simulink model "sampleModel1938"  (R2023a)
settings: Solver=VariableStepAuto  StartTime=0.0  StopTime=10.0  RelTol=1e-3
libraries: hdlsllib x3
settings Model: Creator=user1  LastModifiedBy=user1

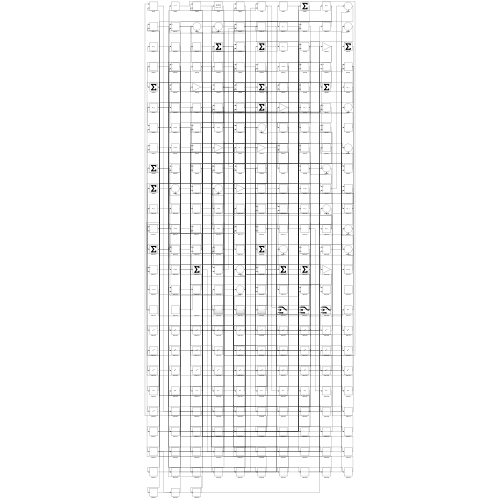
[thumbnail: Simulink's stored preview of the top-level diagram]
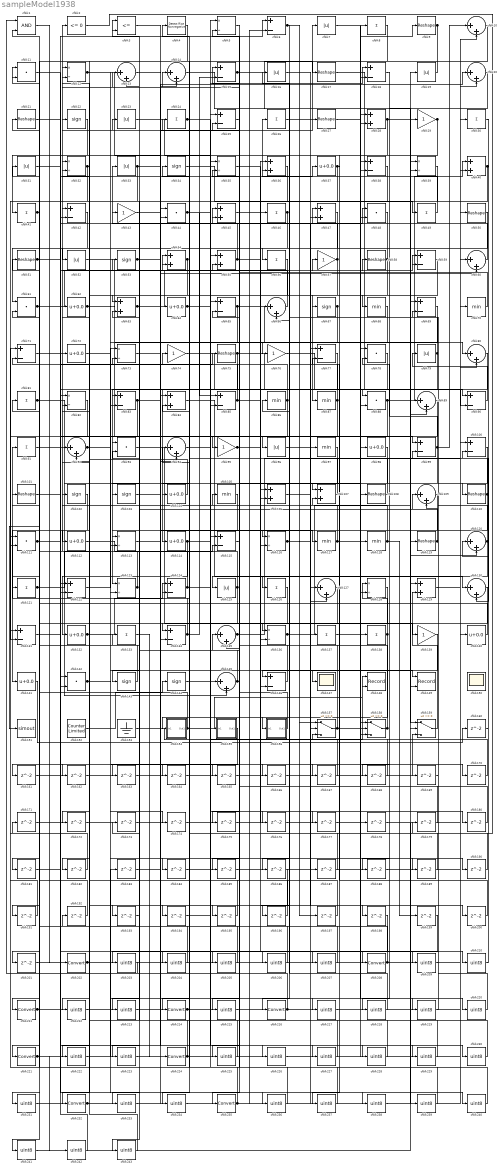
== system sampleModel1938 ==
  cfblk1 : Logic  AllPortsSameDT=off  OutDataTypeStr=boolean
  cfblk{10,13..14,20,60,66,80,89,92,94,109,120,127,130,135,145} (16 alike) : Sum  Inputs=|++
  cfblk{6,15,18,25,38,42,59,65,69,71,77,83,85,90,99..100,115,122,124,131,134,146} (22 alike) : Sum  Inputs=+-
  cfblk{9,17,21,27,50..51,58,75,101,108,110,119} (12 alike) : Reshape
  cfblk{22,34,53,67,102..103,143..144} (8 alike) : Signum
  cfblk{37,62,64,72,98,104,112,114,132,140..141} (11 alike) : Bias  Bias=0.0  SaturateOnIntegerOverflow=off
  cfblk{68,70,86..87,97,105,117..118} (8 alike) : MinMax
  cfblk{28,36,40,45,47,54..55,63,84,106..107,129} (12 alike) : Sum
  cfblk{11,44,48,61,78,88,93,111,142} (9 alike) : DotProduct  OutDataTypeStr=Inherit: Inherit via internal rule
  cfblk{5,12,32,35,39,73,82,113,116,123,128,136} (12 alike) : Product  Inputs=*/  RndMeth=Zero  SaturateOnIntegerOverflow=on
  cfblk{8,24,26,30,41,46,49,56,81,91,121,126,133,137..138} (15 alike) : Sum  Inputs=+
  cfblk{7,16,19,23,31,33,52,79,96,125} (10 alike) : Abs  SaturateOnIntegerOverflow=off
  cfblk{29,43,57,74,76,95,139} (7 alike) : Gain
  cfblk147 : Scope
  cfblk148 : Record  FileSettingsInternal="{\"entries\":[{\"content\":{\"excelSettings\":{\"content\":{},\"type\":\"Streamout.ExcelSettings\"}},\"type\":\"Streamout.FileSettingStorage\",\"uuid\":\"\"}],\"packageUris\":[\"http:\\/\\/schema.mathworks.com\\/mf0\\/streamout_blocks\\/R2020a\"],\"version\":\"1.0\"}"  Layout=[1 1]  SignalsInternal="{\"entries\":[{\"content\":{\"signals\":[{\"content\":{\"blockPath\":[],\"dimensions\":[1],\"domain\":\"\",\"lineColor\":\"#a2142f\",\"plots\":[1],\"port\":1,\"signalID\":5311,\"signalName\":\"XY Graph:1\"},\"type\":\"RecordBlkView.Signal\",\"uuid\":\"\"},{\"content\":{\"blockPath\":[],\"dimensions\":[1],\"domain\":\"\",\"lineColor\":\"#139fff\",\"plots\":[1],\"port\":2,\"signalID\":5314,\"signalName\":\"XY Graph:2\"},\"type\":\"RecordBlkView.Signal\",\"uuid\":\"\"}]},\"type\":\"RecordBlkView.InputSignals\",\"uuid\":\"\"}],\"packageUris\":[\"http:\\/\\/schema.mathworks.com\\/mf0\\/streamout_blocks\\/R2020a\"],\"version\":\"1.0\"}"  VisualizationBindings="{\"xyplotplugin\":{\"info\":[{\"series\":[{\"bindingParametersList\":[{\"parameter\":\"X-Axis\",\"signalID\":5311,\"signalName\":\"XY Graph:1\"},{\"parameter\":\"Y-Axis\",\"signalID\":5314,\"signalName\":\"XY Graph:2\"}],\"seriesID\":33209}],\"subplotID\":1}]}}"  CompatibilityTag=XY  st=-1
  cfblk149 : Record  FileSettingsInternal="{\"entries\":[{\"content\":{\"excelSettings\":{\"content\":{},\"type\":\"Streamout.ExcelSettings\"}},\"type\":\"Streamout.FileSettingStorage\",\"uuid\":\"\"}],\"packageUris\":[\"http:\\/\\/schema.mathworks.com\\/mf0\\/streamout_blocks\\/R2020a\"],\"version\":\"1.0\"}"  Layout=[1 1]  SignalsInternal="{\"entries\":[{\"content\":{\"signals\":[{\"content\":{\"blockPath\":[],\"dimensions\":[1],\"domain\":\"\",\"lineColor\":\"#a2142f\",\"plots\":[1],\"port\":1,\"signalID\":5319,\"signalName\":\"XY Graph:1\"},\"type\":\"RecordBlkView.Signal\",\"uuid\":\"\"},{\"content\":{\"blockPath\":[],\"dimensions\":[1],\"domain\":\"\",\"lineColor\":\"#139fff\",\"plots\":[1],\"port\":2,\"signalID\":5322,\"signalName\":\"XY Graph:2\"},\"type\":\"RecordBlkView.Signal\",\"uuid\":\"\"}]},\"type\":\"RecordBlkView.InputSignals\",\"uuid\":\"\"}],\"packageUris\":[\"http:\\/\\/schema.mathworks.com\\/mf0\\/streamout_blocks\\/R2020a\"],\"version\":\"1.0\"}"  VisualizationBindings="{\"xyplotplugin\":{\"info\":[{\"series\":[{\"bindingParametersList\":[{\"parameter\":\"X-Axis\",\"signalID\":5319,\"signalName\":\"XY Graph:1\"},{\"parameter\":\"Y-Axis\",\"signalID\":5322,\"signalName\":\"XY Graph:2\"}],\"seriesID\":898}],\"subplotID\":1}]}}"  CompatibilityTag=XY  st=-1
  cfblk150 : Scope
      settings: Floating=on
  cfblk151 : ToWorkspace  VariableName=simout  SaveFormat=Timeseries  SampleTime=-1
  cfblk152 : hdlsllib/Sources/Counter Limited  uplimit=7  tsamp=-1
  cfblk153 : Ground
  cfblk154 : Subsystem
      settings: LibrarySourceBlock=|
      | hdlsllib/Ports &
      | Subsystems/Subsystem
  cfblk155 : Subsystem
      settings: LibrarySourceBlock=|
      | hdlsllib/Ports &
      | Subsystems/Subsystem
  cfblk156 : Subsystem
      settings: LibrarySourceBlock=|
      | hdlsllib/Ports &
      | Subsystems/Subsystem
  cfblk157 : Switch  SaturateOnIntegerOverflow=off  InputSameDT=off
  cfblk158 : Switch  SaturateOnIntegerOverflow=off  InputSameDT=off
  cfblk159 : Switch  SaturateOnIntegerOverflow=off  InputSameDT=off
  cfblk{160..201} (42 alike) : Delay  SampleTime=1
  cfblk2 : hdlsllib/Logic and Bit Operations/Compare To Zero  relop=<=  OutDataTypeStr=boolean
  cfblk{202,208,211,214,216,221,224,232,235} (9 alike) : DataTypeConversion  SaturateOnIntegerOverflow=off  RndMeth=Floor
  cfblk{203..207,209..210,212..213,215,217..220,222..223,225..231,233..234,236..243} (33 alike) : DataTypeConversion  OutDataTypeStr=uint8  SaturateOnIntegerOverflow=off  RndMeth=Floor
  cfblk3 : RelationalOperator  Operator=<=  OutDataTypeStr=boolean  InputSameDT=off
  cfblk4 : hdlsllib/Logic and Bit Operations/Detect Rise Nonnegative  vinit=0  OutDataTypeStr=boolean
  wires:
  cfblk116/1 -> cfblk157/1, cfblk190/1
  cfblk17/1 -> cfblk90/1
  cfblk55/1 -> cfblk33/1, cfblk200/1
  cfblk66/1 -> cfblk2/1
  cfblk138/1 -> cfblk128/1, cfblk234/1
  cfblk102/1 -> cfblk141/1
  cfblk118/1 -> cfblk42/1, cfblk199/1
  cfblk46/1 -> cfblk194/1, cfblk195/1
  cfblk19/1 -> cfblk96/1
  cfblk133/1 -> cfblk224/1
  cfblk26/1 -> cfblk7/1
  cfblk80/1 -> cfblk123/1
  cfblk57/1 -> cfblk87/1, cfblk85/2, cfblk45/2
  cfblk153/1 -> cfblk148/1
  cfblk33/1 -> cfblk52/1, cfblk60/2
  cfblk22/1 -> cfblk41/1
  cfblk25/1 -> cfblk235/1
  cfblk24/1 -> cfblk180/1, cfblk207/1
  cfblk41/1 -> cfblk151/1, cfblk11/1
  cfblk84/1 -> cfblk130/1
  cfblk40/1 -> cfblk130/2, cfblk76/1
  cfblk146/1 -> cfblk22/1
  cfblk152/1 -> cfblk144/1
  cfblk51/1 -> cfblk90/2, cfblk59/2
  cfblk127/1 -> cfblk232/1
  cfblk81/1 -> cfblk145/2, cfblk227/1
  cfblk134/1 -> cfblk91/1, cfblk15/2
  cfblk27/1 -> cfblk138/1
  cfblk88/1 -> cfblk40/1, cfblk134/2
  cfblk96/1 -> cfblk48/1
  cfblk156/1(Out1) -> cfblk54/1
  cfblk124/1 -> cfblk3/1, cfblk228/1
  cfblk114/1 -> cfblk132/1, cfblk57/1
  cfblk131/1 -> cfblk72/1
  cfblk4/1 -> cfblk121/1
  cfblk9/1 -> cfblk95/1, cfblk182/1
  cfblk79/1 -> cfblk43/1, cfblk168/1, cfblk243/1
  cfblk8/1 -> cfblk214/1
  cfblk37/1 -> cfblk47/2, cfblk237/1
  cfblk140/1 -> cfblk101/1
  cfblk135/1 -> cfblk30/1, cfblk139/1
  cfblk21/1 -> cfblk99/1
  cfblk87/1 -> cfblk66/2, cfblk215/1
  cfblk48/1 -> cfblk156/1(In1)
  cfblk77/1 -> cfblk93/1
  cfblk129/1 -> cfblk70/1
  cfblk137/1 -> cfblk9/1
  cfblk61/1 -> cfblk58/1, cfblk6/1
  cfblk42/1 -> cfblk61/1
  cfblk157/1 -> cfblk53/1, cfblk219/1
  cfblk154/1(Out1) -> cfblk148/2, cfblk31/1
  cfblk125/1 -> cfblk21/1, cfblk142/2
  cfblk14/1 -> cfblk98/1
  cfblk110/1 -> cfblk113/1, cfblk84/2
  cfblk36/1 -> cfblk103/1
  cfblk12/1 -> cfblk44/2, cfblk165/1
  cfblk104/1 -> cfblk12/1
  cfblk89/1 -> cfblk221/1
  cfblk50/1 -> cfblk216/1
  cfblk58/1 -> cfblk56/1, cfblk147/1
  cfblk117/1 -> cfblk4/1, cfblk16/1, cfblk149/1
  cfblk38/1 -> cfblk211/1
  cfblk99/1 -> cfblk107/1, cfblk78/2, cfblk10/1
  cfblk34/1 -> cfblk49/1
  cfblk28/1 -> cfblk120/2, cfblk122/2
  cfblk93/1 -> cfblk136/1
  cfblk63/1 -> cfblk19/1, cfblk116/2
  cfblk123/1 -> cfblk102/1, cfblk32/1
  cfblk73/1 -> cfblk27/1
  cfblk91/1 -> cfblk128/2
  cfblk75/1 -> cfblk114/1, cfblk158/3, cfblk149/2
  cfblk23/1 -> cfblk155/1(In1)
  cfblk54/1 -> cfblk112/1, cfblk233/1
  cfblk52/1 -> cfblk118/1
  cfblk1/1 -> cfblk202/1
  cfblk132/1 -> cfblk124/1, cfblk146/2
  cfblk121/1 -> cfblk73/1, cfblk83/2
  cfblk136/1 -> cfblk39/1, cfblk198/1
  cfblk49/1 -> cfblk26/1
  cfblk10/1 -> cfblk104/1
  cfblk112/1 -> cfblk115/2
  cfblk119/1 -> cfblk116/1, cfblk23/1
  cfblk35/1 -> cfblk106/1
  cfblk74/1 -> cfblk88/1
  cfblk103/1 -> cfblk20/1
  cfblk120/1 -> cfblk99/2, cfblk125/1
  cfblk122/1 -> cfblk113/2
  cfblk107/1 -> cfblk55/2
  cfblk106/1 -> cfblk77/1
  cfblk101/1 -> cfblk37/1
  cfblk39/1 -> cfblk143/1
  cfblk139/1 -> cfblk146/1
  cfblk67/1 -> cfblk154/1(In1), cfblk134/1
  cfblk142/1 -> cfblk62/1, cfblk174/1
  cfblk62/1 -> cfblk137/1, cfblk184/1, cfblk222/1
  cfblk85/1 -> cfblk51/1, cfblk117/1, cfblk167/1
  cfblk53/1 -> cfblk189/1, cfblk223/1
  cfblk6/1 -> cfblk196/1, cfblk197/1
  cfblk95/1 -> cfblk135/2, cfblk175/1, cfblk210/1
  cfblk56/1 -> cfblk63/1
  cfblk90/1 -> cfblk79/1
  cfblk113/1 -> cfblk64/1
  cfblk59/1 -> cfblk83/1
  cfblk60/1 -> cfblk24/1
  cfblk31/1 -> cfblk42/2
  cfblk76/1 -> cfblk159/1
  cfblk30/1 -> cfblk110/1
  cfblk143/1 -> cfblk81/1
  cfblk64/1 -> cfblk176/1, cfblk177/1
  cfblk158/1 -> cfblk105/1, cfblk12/2
  cfblk86/1 -> cfblk11/2, cfblk181/1
  cfblk83/1 -> cfblk131/2, cfblk230/1
  cfblk29/1 -> cfblk67/1, cfblk126/1
  cfblk45/1 -> cfblk46/1
  cfblk20/1 -> cfblk68/1
  cfblk92/1 -> cfblk172/1, cfblk206/1
  cfblk32/1 -> cfblk111/2, cfblk161/1, cfblk162/1
  cfblk108/1 -> cfblk54/2
  cfblk159/1 -> cfblk129/2
  cfblk145/1 -> cfblk65/2, cfblk73/2, cfblk45/1
  cfblk144/1 -> cfblk59/1
  cfblk70/1 -> cfblk15/1
  cfblk111/1 -> cfblk75/1, cfblk47/1
  cfblk65/1 -> cfblk80/1, cfblk123/2, cfblk6/2
  cfblk3/1 -> cfblk14/2
  cfblk68/1 -> cfblk158/2
  cfblk100/1 -> cfblk208/1
  cfblk44/1 -> cfblk85/1, cfblk18/1, cfblk166/1
  cfblk115/1 -> cfblk35/2
  cfblk15/1 -> cfblk119/1, cfblk17/1
  cfblk141/1 -> cfblk160/1
  cfblk160/1 -> cfblk120/1
  cfblk161/1 -> cfblk39/2
  cfblk162/1 -> cfblk106/2
  cfblk130/1 -> cfblk163/1
  cfblk163/1 -> cfblk35/1
  cfblk105/1 -> cfblk164/1
  cfblk165/1 -> cfblk129/1
  cfblk166/1 -> cfblk159/3
  cfblk167/1 -> cfblk157/3
  cfblk168/1 -> cfblk115/1
  cfblk169/1 -> cfblk69/2
  cfblk43/1 -> cfblk170/1
  cfblk170/1 -> cfblk157/2
  cfblk171/1 -> cfblk28/2
  cfblk172/1 -> cfblk136/2
  cfblk173/1 -> cfblk3/2
  cfblk174/1 -> cfblk20/2
  cfblk175/1 -> cfblk48/2
  cfblk176/1 -> cfblk159/2
  cfblk177/1 -> cfblk77/2
  cfblk7/1 -> cfblk178/1
  cfblk2/1 -> cfblk179/1
  cfblk179/1 -> cfblk36/1
  cfblk180/1 -> cfblk135/1
  cfblk182/1 -> cfblk131/1
  cfblk183/1 -> cfblk44/1
  cfblk184/1 -> cfblk80/2
  cfblk128/1 -> cfblk185/1
  cfblk185/1 -> cfblk88/2
  cfblk97/1 -> cfblk186/1
  cfblk16/1 -> cfblk187/1
  cfblk187/1 -> cfblk55/1
  cfblk18/1 -> cfblk188/1
  cfblk188/1 -> cfblk40/2
  cfblk189/1 -> cfblk14/1
  cfblk190/1 -> cfblk124/2
  cfblk155/1(Out1) -> cfblk191/1
  cfblk191/1 -> cfblk111/1
  cfblk192/1 -> cfblk61/2
  cfblk78/1 -> cfblk193/1
  cfblk193/1 -> cfblk93/2
  cfblk194/1 -> cfblk145/1
  cfblk195/1 -> cfblk32/2
  cfblk196/1 -> cfblk65/1
  cfblk197/1 -> cfblk63/2
  cfblk200/1 -> cfblk107/2
  cfblk126/1 -> cfblk201/1
  cfblk201/1 -> cfblk29/1
  cfblk202/1 -> cfblk140/1, cfblk240/1
  cfblk198/1 -> cfblk203/1
  cfblk203/1 -> cfblk1/1
  cfblk199/1 -> cfblk204/1
  cfblk204/1 -> cfblk1/2
  cfblk5/1 -> cfblk205/1
  cfblk205/1 -> cfblk171/1
  cfblk206/1 -> cfblk5/1
  cfblk207/1 -> cfblk5/2
  cfblk208/1 -> cfblk122/1, cfblk86/1
  cfblk181/1 -> cfblk209/1
  cfblk209/1 -> cfblk100/1
  cfblk210/1 -> cfblk100/2
  cfblk211/1 -> cfblk108/1, cfblk28/1
  cfblk186/1 -> cfblk212/1
  cfblk212/1 -> cfblk38/1
  cfblk69/1 -> cfblk213/1
  cfblk213/1 -> cfblk38/2
  cfblk214/1 -> cfblk18/2, cfblk158/1
  cfblk215/1 -> cfblk8/1
  cfblk216/1 -> cfblk173/1, cfblk142/1
  cfblk72/1 -> cfblk217/1
  cfblk217/1 -> cfblk50/1
  cfblk109/1 -> cfblk218/1
  cfblk218/1 -> cfblk36/2
  cfblk219/1 -> cfblk109/1
  cfblk164/1 -> cfblk220/1
  cfblk220/1 -> cfblk109/2
  cfblk221/1 -> cfblk183/1, cfblk84/1, cfblk242/1
  cfblk222/1 -> cfblk89/1
  cfblk223/1 -> cfblk89/2
  cfblk224/1 -> cfblk192/1, cfblk10/2, cfblk74/1
  cfblk98/1 -> cfblk225/1
  cfblk225/1 -> cfblk133/1
  cfblk13/1 -> cfblk226/1
  cfblk226/1 -> cfblk78/1
  cfblk227/1 -> cfblk13/1
  cfblk228/1 -> cfblk13/2
  cfblk94/1 -> cfblk229/1
  cfblk229/1 -> cfblk92/1
  cfblk230/1 -> cfblk94/1
  cfblk47/1 -> cfblk231/1
  cfblk231/1 -> cfblk94/2
  cfblk232/1 -> cfblk92/2, cfblk97/1
  cfblk233/1 -> cfblk127/1
  cfblk234/1 -> cfblk127/2
  cfblk235/1 -> cfblk60/1, cfblk66/1, cfblk34/1
  cfblk11/1 -> cfblk236/1
  cfblk236/1 -> cfblk25/1
  cfblk237/1 -> cfblk25/2
  cfblk71/1 -> cfblk238/1
  cfblk238/1 -> cfblk69/1
  cfblk178/1 -> cfblk239/1
  cfblk239/1 -> cfblk71/1
  cfblk240/1 -> cfblk71/2
  cfblk82/1 -> cfblk241/1
  cfblk241/1 -> cfblk169/1
  cfblk242/1 -> cfblk82/1
  cfblk243/1 -> cfblk82/2

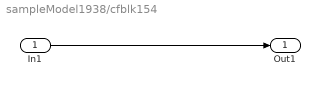
== system sampleModel1938/cfblk154 ==
  In1 : Inport
  Out1 : Outport
  wires:
  In1/1 -> Out1/1

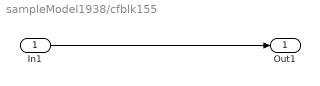
== system sampleModel1938/cfblk155 ==
  In1 : Inport
  Out1 : Outport
  wires:
  In1/1 -> Out1/1

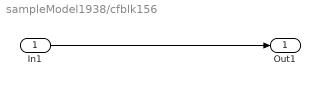
== system sampleModel1938/cfblk156 ==
  In1 : Inport
  Out1 : Outport
  wires:
  In1/1 -> Out1/1
